simulink model "PIDWirings"  (R2018b)
settings: Solver=VariableStepAuto  StartTime=0.0  StopTime=10.0  RelTol=1e-3
settings Model: Creator=y.briere  LastModifiedBy=y.briere

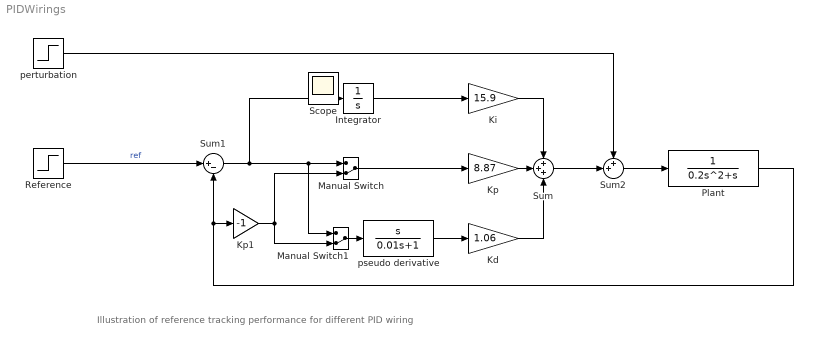
== system PIDWirings ==
  note: Illustration of reference tracking performance for different PID wiring
  Integrator : Integrator
  Kd : Gain  Gain=1.06
  Ki : Gain  Gain=15.9
  Kp : Gain  Gain=8.87
  Kp1 : Gain  Gain=-1
  Manual Switch : ManualSwitch  CurrentSetting=0
  Manual Switch1 : ManualSwitch  CurrentSetting=0
  Plant : TransferFcn  Denominator=[0.2 1 0]
  Reference : Step  SampleTime=0
  Sum : Sum  Inputs=+++
  Sum1 : Sum  Inputs=|+-
  Sum2 : Sum  Inputs=++|
  perturbation : Step  Time=5  After=0.2  SampleTime=0
  pseudo derivative : TransferFcn  Numerator=[1 0]  Denominator=[0.01 1]
  Scope : Scope
  wires:
  Kp/1 -> Sum/2
  Plant/1 -> Sum1/2, Kp1/1
  Sum1/1 -> Manual Switch/1, Manual Switch1/1, Integrator/1
  Ki/1 -> Sum/1
  Reference/1 -> Sum1/1  "ref"
  Manual Switch/1 -> Kp/1
  Kp1/1 -> Manual Switch1/2, Manual Switch/2
  Kd/1 -> Sum/3
  Integrator/1 -> Ki/1
  pseudo derivative/1 -> Kd/1
  Sum/1 -> Sum2/2
  Sum2/1 -> Plant/1
  perturbation/1 -> Sum2/1
  Manual Switch1/1 -> pseudo derivative/1
